simulink model "Slide_SLIPControl_Uneven"  (R2020b)
settings: Solver=VariableStepAuto  StartTime=0.0  StopTime=10  FixedStep=0.01  RelTol=1e-3
undefined symbols (not defined in the file or in its folder): B, Feet, T1, T10, T11, T2, T3, T4, T5, T6, T7, T8, T9, Thigh, Torso, X, Y, Z
libraries: sm_lib x159, nesl_utility x22, simulink x1
(part 1 of 3)
settings Model: Creator=chainplain  LastModifiedBy=chainplain

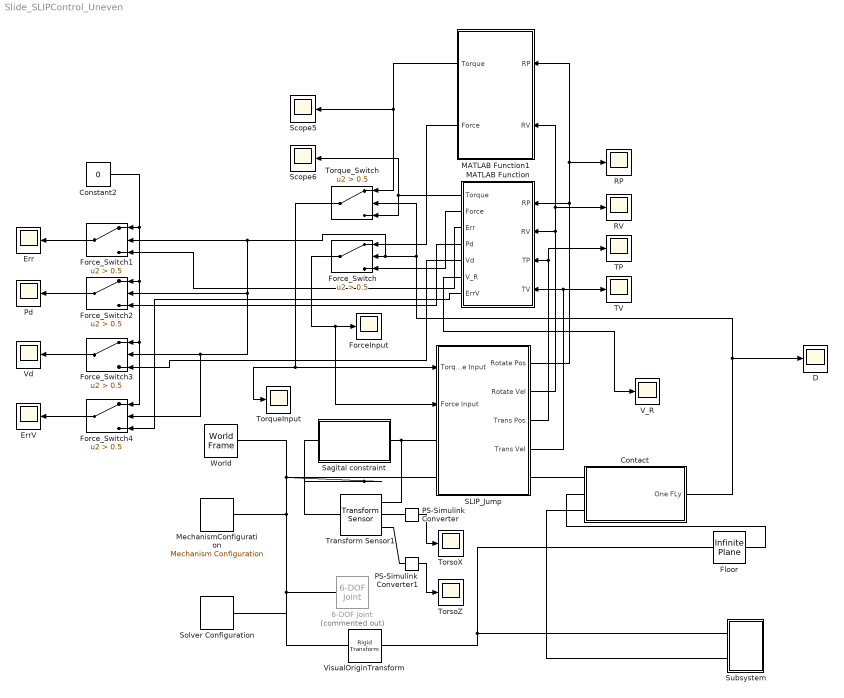
== system Slide_SLIPControl_Uneven ==
  6-DOF Joint : sm_lib/Joints/6-DOF Joint  Commented=on  JointMode=Normal  SenseConstraintForce=off  SenseConstraintForceX=off  SenseConstraintForceY=off  SenseConstraintForceZ=off  SenseConstraintTorque=off  SenseConstraintTorqueX=off  SenseConstraintTorqueY=off  SenseConstraintTorqueZ=off  SenseTotalForce=off  SenseTotalForceX=off  SenseTotalForceY=off  SenseTotalForceZ=off  SenseTotalTorque=off  SenseTotalTorqueX=off  SenseTotalTorqueY=off  SenseTotalTorqueZ=off  CompositeWrenchDir=FollowerOnBase  CompositeWrenchFrame=BaseFrame  PxEquilibriumPosition=0  PxEquilibriumPositionUnits=m  PxSpringStiffness=0  PxSpringStiffnessUnits=N/m  PxDampingCoefficient=0  PxDampingCoefficientUnits=N/(m/s)  PxTorqueActuationMode=NoTorque  PxMotionActuationMode=ComputedMotion  PxSensePosition=off  PxSenseVelocity=off  PxSenseAcceleration=off  PxSenseTorqueForce=off  PxSenseLowerLimitTorqueForce=off  PxSenseUpperLimitTorqueForce=off  PxLowerLimitSpecify=off  PxLowerLimitBound=-1  PxLowerLimitBoundUnits=m  PxLowerLimitStiffness=1e6  PxLowerLimitStiffnessUnits=N/m  PxLowerLimitDamping=1e3  PxLowerLimitDampingUnits=N/(m/s)  PxLowerLimitTransitionRegionWidth=1e-4  PxLowerLimitTransitionRegionWidthUnits=m  PxUpperLimitSpecify=off  PxUpperLimitBound=1  PxUpperLimitBoundUnits=m  PxUpperLimitStiffness=1e6  PxUpperLimitStiffnessUnits=N/m  PxUpperLimitDamping=1e3  PxUpperLimitDampingUnits=N/(m/s)  PxUpperLimitTransitionRegionWidth=1e-4  PxUpperLimitTransitionRegionWidthUnits=m  PxPositionTargetSpecify=off  PxPositionTargetPriority=High  PxPositionTargetValue=0  PxPositionTargetValueUnits=m  PxVelocityTargetSpecify=off  PxVelocityTargetPriority=High  PxVelocityTargetValue=0  PxVelocityTargetValueUnits=m/s  PyEquilibriumPosition=0  PyEquilibriumPositionUnits=m  PySpringStiffness=0  PySpringStiffnessUnits=N/m  PyDampingCoefficient=0  PyDampingCoefficientUnits=N/(m/s)  PyTorqueActuationMode=NoTorque  PyMotionActuationMode=ComputedMotion  PySensePosition=off  PySenseVelocity=off  PySenseAcceleration=off  PySenseTorqueForce=off  PySenseLowerLimitTorqueForce=off  PySenseUpperLimitTorqueForce=off  PyLowerLimitSpecify=off  PyLowerLimitBound=-1  PyLowerLimitBoundUnits=m  PyLowerLimitStiffness=1e6  PyLowerLimitStiffnessUnits=N/m  PyLowerLimitDamping=1e3  PyLowerLimitDampingUnits=N/(m/s)  PyLowerLimitTransitionRegionWidth=1e-4  PyLowerLimitTransitionRegionWidthUnits=m  PyUpperLimitSpecify=off  PyUpperLimitBound=1  PyUpperLimitBoundUnits=m  PyUpperLimitStiffness=1e6  PyUpperLimitStiffnessUnits=N/m  PyUpperLimitDamping=1e3  PyUpperLimitDampingUnits=N/(m/s)  PyUpperLimitTransitionRegionWidth=1e-4  PyUpperLimitTransitionRegionWidthUnits=m  PyPositionTargetSpecify=off  PyPositionTargetPriority=High  PyPositionTargetValue=0  PyPositionTargetValueUnits=m  PyVelocityTargetSpecify=off  PyVelocityTargetPriority=High  PyVelocityTargetValue=0  PyVelocityTargetValueUnits=m/s  PzEquilibriumPosition=0  PzEquilibriumPositionUnits=m  PzSpringStiffness=0  PzSpringStiffnessUnits=N/m  PzDampingCoefficient=0  PzDampingCoefficientUnits=N/(m/s)  PzTorqueActuationMode=NoTorque  PzMotionActuationMode=ComputedMotion  PzSensePosition=off  PzSenseVelocity=off  PzSenseAcceleration=off  PzSenseTorqueForce=off  PzSenseLowerLimitTorqueForce=off  PzSenseUpperLimitTorqueForce=off  PzLowerLimitSpecify=off  PzLowerLimitBound=-1  PzLowerLimitBoundUnits=m  PzLowerLimitStiffness=1e6  PzLowerLimitStiffnessUnits=N/m  PzLowerLimitDamping=1e3  PzLowerLimitDampingUnits=N/(m/s)  PzLowerLimitTransitionRegionWidth=1e-4  PzLowerLimitTransitionRegionWidthUnits=m  PzUpperLimitSpecify=off  PzUpperLimitBound=1  PzUpperLimitBoundUnits=m  PzUpperLimitStiffness=1e6  PzUpperLimitStiffnessUnits=N/m  PzUpperLimitDamping=1e3  PzUpperLimitDampingUnits=N/(m/s)  PzUpperLimitTransitionRegionWidth=1e-4  PzUpperLimitTransitionRegionWidthUnits=m  PzPositionTargetSpecify=off  PzPositionTargetPriority=High  PzPositionTargetValue=0  PzPositionTargetValueUnits=m  PzVelocityTargetSpecify=off  PzVelocityTargetPriority=High  PzVelocityTargetValue=0  PzVelocityTargetValueUnits=m/s  SphDefPosRotationMethod=None  SphDefPosRotationAngleUnits=deg  SphDefPosRotationStandardAxis=+Z  SphDefPosRotationAngle=0.0  SphDefPosRotationArbitraryAxis=[0 0 1]  SphDefPosFollAlignAxisA=+X  SphDefPosBaseAlignAxisA=+Y  SphDefPosFollAlignAxisB=+Y  SphDefPosBaseAlignAxisB=+Z  SphDefPosRotationSequenceAxes=FollowerAxes  SphDefPosRotationSequence=XYX  SphDefPosRotationSequenceAngles=[0 0 0]  SphDefPosRotationSequenceAnglesUnits=deg  SphDefPosRotationMatrix=[1 0 0; 0 1 0; 0 0 1]  SphEqPosRotationMethod=None  SphEqPosRotationAngleUnits=deg  SphEqPosRotationStandardAxis=+Z  SphEqPosRotationAngle=0.0  SphEqPosRotationArbitraryAxis=[0 0 1]  SphEqPosFollAlignAxisA=+X  SphEqPosBaseAlignAxisA=+Y  SphEqPosFollAlignAxisB=+Y  SphEqPosBaseAlignAxisB=+Z  SphEqPosRotationSequenceAxes=FollowerAxes  SphEqPosRotationSequence=XYX  SphEqPosRotationSequenceAngles=[0 0 0]  SphEqPosRotationSequenceAnglesUnits=deg  SphEqPosRotationMatrix=[1 0 0; 0 1 0; 0 0 1]  SphSpringStiffness=0  SphSpringStiffnessUnits=N*m/deg  SphDampingCoefficient=0  SphDampingCoefficientUnits=N*m/(deg/s)  SphActuateTorqueX=off  SphActuateTorqueY=off  SphActuateTorqueZ=off  SphActuateTorque=off  SphTorqueActuationMode=NoTorque  SphMotionActuationMode=ComputedMotion  SphActuationFrame=BaseFrame  SphSensePosition=off  SphSenseVelocityX=off  SphSenseVelocityY=off  SphSenseVelocityZ=off  SphSenseVelocity=off  SphSenseAccelerationX=off  SphSenseAccelerationY=off  SphSenseAccelerationZ=off  SphSenseAcceleration=off  SphSenseTorqueX=off  SphSenseTorqueY=off  SphSenseTorqueZ=off  SphSenseTorqueForce=off  SphSenseLowerLimitTorqueMag=off  SphSenseUpperLimitTorqueMag=off  SphSensingFrame=BaseFrame  SphLowerLimitSpecify=off  SphLowerLimitBound=15  SphLowerLimitBoundUnits=deg  SphLowerLimitStiffness=1e4  SphLowerLimitStiffnessUnits=N*m/deg  SphLowerLimitDamping=10  SphLowerLimitDampingUnits=N*m/(deg/s)  SphLowerLimitTransitionRegionWidth=0.1  SphLowerLimitTransitionRegionWidthUnits=deg  SphUpperLimitSpecify=off  SphUpperLimitBound=45  SphUpperLimitBoundUnits=deg  SphUpperLimitStiffness=1e4  SphUpperLimitStiffnessUnits=N*m/deg  SphUpperLimitDamping=10  SphUpperLimitDampingUnits=N*m/(deg/s)  SphUpperLimitTransitionRegionWidth=0.1  SphUpperLimitTransitionRegionWidthUnits=deg  SphPositionTargetRotationMethod=None  SphPositionTargetRotationAngleUnits=deg  SphPositionTargetRotationStandardAxis=+Z  SphPositionTargetRotationAngle=0.0  SphPositionTargetRotationArbitraryAxis=[0 0 1]  SphPositionTargetFollAlignAxisA=+X  SphPositionTargetBaseAlignAxisA=+Y  SphPositionTargetFollAlignAxisB=+Y  SphPositionTargetBaseAlignAxisB=+Z  SphPositionTargetRotationSequenceAxes=FollowerAxes  SphPositionTargetRotationSequence=XYX  SphPositionTargetRotationSequenceAngles=[0 0 0]  SphPositionTargetRotationSequenceAnglesUnits=deg  SphPositionTargetRotationMatrix=[1 0 0; 0 1 0; 0 0 1]  SphPositionTargetSpecify=off  SphPositionTargetPriority=High  SphVelocityTargetValue=[0 0 0]  SphVelocityTargetValueUnits=deg/s  SphVelocityTargetSpecify=off  SphVelocityTargetPriority=High  SphVelocityTargetInFollowerFrame=on
  Constant2 : Constant  Value=0
  Contact : Subsystem  mask{Stiff=1e6, Damp=1e3, Trans=1e-4, StaticF=0.750, DynamicF=0.500, CriticalV=1e-4}
      mask prompts: Stiff "Contact Stiffness"; Damp "Contact Damping"; Trans "Contact TransRegion"; StaticF "Contact Static Friction"; DynamicF "Contact Dynamic Friction"; CriticalV "Contact Critical Velocity"
      mask DialogControl ContactGroupVar Prompt: Contact
  D : Scope
  Err : Scope
  ErrV : Scope
  Floor : sm_lib/Curves and Surfaces/Infinite Plane  GraphicType=Rectangle  GraphicPlaneWidth=100  GraphicPlaneWidthUnits=m  GraphicPlaneHeight=1  GraphicPlaneHeightUnits=m  GraphicVisPropType=SimpleVisualProperties  GraphicDiffuseColor=[0.5 0.5 0.5]  GraphicOpacity=1  GraphicSpecularColor=[0.5 0.5 0.5 1.0]  GraphicAmbientColor=[0.15 0.15 0.15 1.0]  GraphicEmissiveColor=[0.0 0.0 0.0 1.0]  GraphicShininess=75
  ForceInput : Scope
  Force_Switch{,1..4} (5 alike) : Switch  Criteria=u2 > Threshold  Threshold=0.5
  MATLAB Function : MATLAB Function  TreatAsAtomicUnit=on
  MATLAB Function1 : MATLAB Function  TreatAsAtomicUnit=on
  MechanismConfiguration : sm_lib/Utilities/Mechanism Configuration  UniformGravity=Constant  GravityVector=[0 0 -9.80665]  GravityVectorUnits=m/s^2  GravityUnits=m/s^2  LinearizationDelta=0.001  JointModeTransitionNonlinearIterations=2
  PS-Simulink Converter : nesl_utility/PS-Simulink Converter  PhysicalDomain=network_engine_domain  SubClassName=ps_output  LeftPortType=input  RightPortType=output  PseudoPeriodic=off  Frequencies=[]  Unit=inherit  AffineConversion=off
  PS-Simulink Converter1 : nesl_utility/PS-Simulink Converter  PhysicalDomain=network_engine_domain  SubClassName=ps_output  LeftPortType=input  RightPortType=output  PseudoPeriodic=off  Frequencies=[]  Unit=inherit  AffineConversion=off
  Pd : Scope
  RP : Scope
  RV : Scope
  SLIP_Jump : Subsystem
      mask Display: image('SlipFig.png'); % Use "Edit Image" on toolstrip to change.
  Sagital constraint : Subsystem
  Scope5 : Scope
  Scope6 : Scope
  Solver Configuration : nesl_utility/Solver Configuration  PhysicalDomain=network_engine_domain  SubClassName=solver  LeftPortType=input  RightPortType=generic  Tones=[]  Harmonics=[]  SimulateNoise=off  Profile=off  UseLocalSampling=off  EnableSwitchedLinearOptims=on  FrequencyDomain=off  UseCCode=off  RelTol=0.001  AbsTol=1e-06  MinStep=1e-09  ToWorkspace=off  RevertToSquareIcSolve=off  NumHomotopyIterations=100  PhasorMode=off  PhasorModeNumHarmonics=1  DoDC=off  ResidualTolerance=1e-09  UseLocalSolver=off  LocalSolverChoice=NE_BACKWARD_EULER_ADVANCER  LocalSolverSampleTime=0.001  DoFixedCost=off  MaxNonlinIter=3  MaxModeIter=2  ComputeImpulses=off  ImpulseIterations=2  LinearAlgebra=auto  EquationFormulation=NE_TIME_EF  DelaysMemoryBudget=1024  AutomaticFiltering=on  FilteringTimeConstant=0.001  PartitionStorageMethod=AS_NEEDED  PartitionMemoryBudget=1024  PartitionMethod=ROBUST
  Subsystem : Subsystem
  TP : Scope
  TV : Scope
  TorqueInput : Scope
  Torque_Switch : Switch  Criteria=u2 > Threshold  Threshold=0.5
  TorsoX : Scope
  TorsoZ : Scope
  Transform Sensor1 : sm_lib/Frames and Transforms/Transform Sensor  MeasurementFrame=World  SenseAngle=off  SenseAxis=off  SenseAngle1=off  SenseAngle2=off  SenseAngle3=off  SenseQ=off  SenseR=off  SenseOmegaX=off  SenseOmegaY=off  SenseOmegaZ=off  SenseOmega1=off  SenseOmega2=off  SenseOmega3=off  SenseQDot=off  SenseRDot=off  SenseAlphaX=off  SenseAlphaY=off  SenseAlphaZ=off  SenseAlpha1=off  SenseAlpha2=off  SenseAlpha3=off  SenseQDDot=off  SenseRDDot=off  SenseX=on  SenseY=off  SenseZ=on  SenseRad=off  SenseAzim=off  SenseDist=off  SenseInc=off  SenseXDot=off  SenseYDot=off  SenseZDot=off  SenseRadDot=off  SenseAzimDot=off  SenseDistDot=off  SenseIncDot=off  SenseXDDot=off  SenseYDDot=off  SenseZDDot=off  SenseRadDDot=off  SenseAzimDDot=off  SenseDistDDot=off  SenseIncDDot=off
  V_R : Scope
  Vd : Scope
  VisualOriginTransform : sm_lib/Frames and Transforms/Rigid Transform  TranslationMethod=Cartesian  TranslationStandardOffset=0  TranslationLengthUnit=m  TranslationStandardAxis=+Z  TranslationCartesianOffset=[0, 0.3, -0.7]  TranslationROffset=0  TranslationROffsetUnits=m  TranslationZOffset=0  TranslationZOffsetUnits=m  TranslationThetaOffset=0  TranslationThetaOffsetUnits=deg  RotationMethod=RotationSequence  RotationAngleUnits=deg  RotationStandardAxis=+Z  RotationAngle=0.0  RotationArbitraryAxis=[0 0 1]  FollAlignAxisA=+X  BaseAlignAxisA=+Y  FollAlignAxisB=+Y  BaseAlignAxisB=+Z  RotationSequenceAxes=BaseAxes  RotationSequence=XYZ  RotationSequenceAngles=[0, 0, 0]  RotationSequenceAnglesUnits=rad  RotationMatrix=[1 0 0; 0 1 0; 0 0 1]
  World : sm_lib/Frames and Transforms/World Frame
  wires:
  SLIP_Jump/1(Rotate Pos) -> RP/1, MATLAB Function1/1(RP), MATLAB Function/1(RP)
  SLIP_Jump/2(Rotate Vel) -> RV/1, MATLAB Function1/2(RV), MATLAB Function/2(RV)
  SLIP_Jump/3(Trans Pos) -> TP/1, MATLAB Function/3(TP)
  SLIP_Jump/4(Trans Vel) -> TV/1, MATLAB Function/4(TV)
  MATLAB Function1/1(Torque) -> Torque_Switch/1, Scope5/1
  MATLAB Function1/2(Force) -> Force_Switch/1
  Force_Switch/1 -> SLIP_Jump/2(Force Input), ForceInput/1
  Torque_Switch/1 -> TorqueInput/1, SLIP_Jump/1(Torque Input)
  MATLAB Function/1(Torque) -> Scope6/1, Torque_Switch/3
  MATLAB Function/2(Force) -> Force_Switch/3
  MATLAB Function/3(Err) -> Force_Switch1/3
  Constant2/1 -> Force_Switch4/1, Force_Switch3/1, Force_Switch2/1, Force_Switch1/1
  Force_Switch1/1 -> Err/1
  MATLAB Function/4(Pd) -> Force_Switch2/3
  Contact/1(One FLy) -> Force_Switch4/2, Force_Switch3/2, Force_Switch2/2, Force_Switch1/2, Force_Switch/2, Torque_Switch/2, D/1
  Force_Switch2/1 -> Pd/1
  Force_Switch3/1 -> Vd/1
  Force_Switch4/1 -> ErrV/1
  MATLAB Function/5(Vd) -> Force_Switch3/3
  MATLAB Function/7(ErrV) -> Force_Switch4/3
  PS-Simulink Converter/1 -> TorsoX/1
  PS-Simulink Converter1/1 -> TorsoZ/1
  MATLAB Function/6(V_R) -> V_R/1
  connections:
  MechanismConfiguration/RConn1 -- Transform Sensor1/LConn1 -- Sagital constraint/LConn1 -- World/RConn1 -- SLIP_Jump/LConn2 -- VisualOriginTransform/LConn1 -- Solver Configuration/RConn1 -- 6-DOF Joint/LConn1
  VisualOriginTransform/RConn1 -- Floor/LConn1 -- Subsystem/LConn1
  SLIP_Jump/RConn1 -- Contact/LConn1
  Contact/LConn2 -- Floor/RConn1
  Sagital constraint/RConn1 -- Transform Sensor1/RConn1 -- SLIP_Jump/LConn1
  Contact/LConn3 -- Subsystem/LConn2
  PS-Simulink Converter/LConn1 -- Transform Sensor1/RConn2
  Transform Sensor1/RConn3 -- PS-Simulink Converter1/LConn1

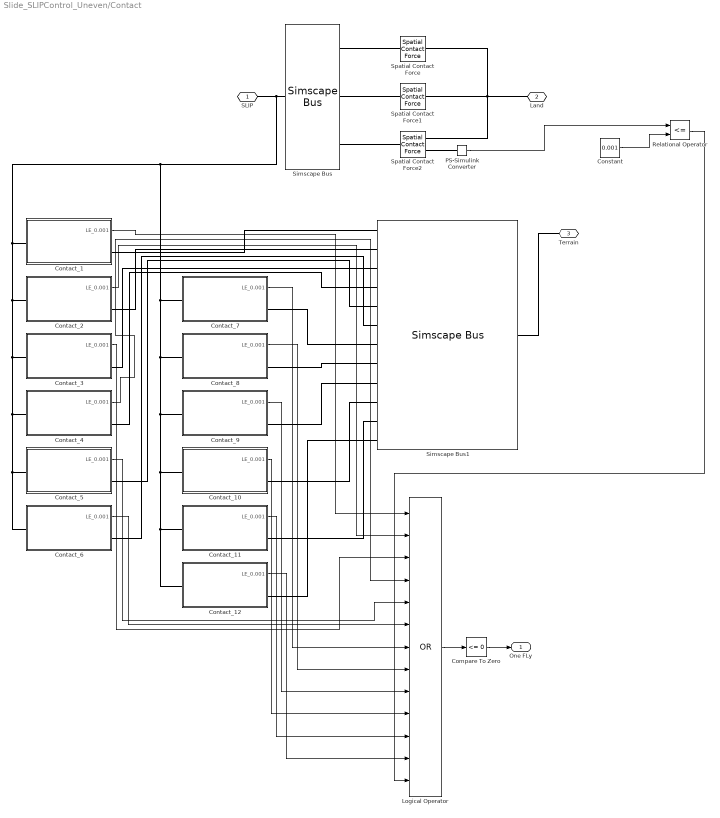
== system Slide_SLIPControl_Uneven/Contact ==
  Compare To Zero : simulink/Logic and Bit Operations/Compare To Zero  relop=<=  OutDataTypeStr=boolean
  Constant : Constant  Value=0.001
  Contact_1 : Subsystem
  Contact_10 : Subsystem
  Contact_11 : Subsystem
  Contact_12 : Subsystem
  Contact_2 : Subsystem
  Contact_3 : Subsystem
  Contact_4 : Subsystem
  Contact_5 : Subsystem
  Contact_6 : Subsystem
  Contact_7 : Subsystem
  Contact_8 : Subsystem
  Contact_9 : Subsystem
  Logical Operator : Logic  Operator=OR  Inputs=13  AllPortsSameDT=off  OutDataTypeStr=boolean
  PS-Simulink Converter : nesl_utility/PS-Simulink Converter  PhysicalDomain=network_engine_domain  SubClassName=ps_output  LeftPortType=input  RightPortType=output  PseudoPeriodic=off  Frequencies=[]  Unit=inherit  AffineConversion=off
  Relational Operator : RelationalOperator  Operator=<=  OutDataTypeStr=boolean  RndMeth=Simplest
  Simscape Bus : SimscapeBus  HierarchyStrings=Torso;Thigh;Feet
  Simscape Bus1 : SimscapeBus  HierarchyStrings=B;T1;T2;T3;T4;T5;T6;T7;T8;T9;T10;T11
  Spatial Contact Force : sm_lib/Forces and Torques/Spatial Contact Force  CoefficientOfDynamicFriction=DynamicF  CoefficientOfStaticFriction=StaticF  NormalDamping=Damp  NormalDampingUnits=N/(m/s)  NormalStiffness=Stiff  NormalStiffnessUnits=N/m  FrictionalCriticalVelocity=CriticalV  FrictionalCriticalVelocityUnits=m/s  ZeroCrossDetectContactStartAndEnd=off  SenseFrictionalForceMagnitude=off  SenseNormalForceMagnitude=off  SenseSeparationDistance=off  NormalTransitionRegionWidth=Trans  NormalTransitionRegionWidthUnits=m  FrictionType=SmoothStickSlip
  Spatial Contact Force1 : sm_lib/Forces and Torques/Spatial Contact Force  CoefficientOfDynamicFriction=DynamicF  CoefficientOfStaticFriction=StaticF  NormalDamping=Damp  NormalDampingUnits=N/(m/s)  NormalStiffness=Stiff  NormalStiffnessUnits=N/m  FrictionalCriticalVelocity=CriticalV  FrictionalCriticalVelocityUnits=m/s  ZeroCrossDetectContactStartAndEnd=off  SenseFrictionalForceMagnitude=off  SenseNormalForceMagnitude=off  SenseSeparationDistance=off  NormalTransitionRegionWidth=Trans  NormalTransitionRegionWidthUnits=m  FrictionType=SmoothStickSlip
  Spatial Contact Force2 : sm_lib/Forces and Torques/Spatial Contact Force  CoefficientOfDynamicFriction=DynamicF  CoefficientOfStaticFriction=StaticF  NormalDamping=Damp  NormalDampingUnits=N/(m/s)  NormalStiffness=Stiff  NormalStiffnessUnits=N/m  FrictionalCriticalVelocity=CriticalV  FrictionalCriticalVelocityUnits=m/s  ZeroCrossDetectContactStartAndEnd=off  SenseFrictionalForceMagnitude=off  SenseNormalForceMagnitude=off  SenseSeparationDistance=on  NormalTransitionRegionWidth=Trans  NormalTransitionRegionWidthUnits=m  FrictionType=SmoothStickSlip
  SLIP : PMIOPort  Side=Left
  Land : PMIOPort  Port=2  Side=Left
  Terrain : PMIOPort  Port=3  Side=Left
  One FLy : Outport
  wires:
  Contact_1/1(LE_0.001) -> Logical Operator/1
  Contact_2/1(LE_0.001) -> Logical Operator/2
  Contact_3/1(LE_0.001) -> Logical Operator/3
  Contact_4/1(LE_0.001) -> Logical Operator/4
  Contact_5/1(LE_0.001) -> Logical Operator/5
  Contact_6/1(LE_0.001) -> Logical Operator/6
  Contact_7/1(LE_0.001) -> Logical Operator/7
  Contact_8/1(LE_0.001) -> Logical Operator/8
  Contact_9/1(LE_0.001) -> Logical Operator/9
  Contact_10/1(LE_0.001) -> Logical Operator/10
  Contact_11/1(LE_0.001) -> Logical Operator/11
  Contact_12/1(LE_0.001) -> Logical Operator/12
  Relational Operator/1 -> Logical Operator/13
  PS-Simulink Converter/1 -> Relational Operator/1
  Constant/1 -> Relational Operator/2
  Compare To Zero/1 -> One FLy/1
  Logical Operator/1 -> Compare To Zero/1
  connections:
  SLIP/RConn1 -- Contact_12/LConn1 -- Contact_11/LConn1 -- Contact_10/LConn1 -- Contact_9/LConn1 -- Contact_8/LConn1 -- Contact_7/LConn1 -- Contact_6/LConn1 -- Contact_5/LConn1 -- Contact_4/LConn1 -- Contact_3/LConn1 -- Contact_2/LConn1 -- Contact_1/LConn1 -- Simscape Bus/RConn1
  Spatial Contact Force/LConn1 -- Simscape Bus/LConn1
  Simscape Bus/LConn2 -- Spatial Contact Force1/LConn1
  Simscape Bus/LConn3 -- Spatial Contact Force2/LConn1
  Spatial Contact Force/RConn1 -- Land/RConn1 -- Spatial Contact Force1/RConn1 -- Spatial Contact Force2/RConn1
  PS-Simulink Converter/LConn1 -- Spatial Contact Force2/RConn2
  Simscape Bus1/RConn1 -- Terrain/RConn1
  Contact_1/RConn1 -- Simscape Bus1/LConn1
  Contact_2/RConn1 -- Simscape Bus1/LConn2
  Contact_3/RConn1 -- Simscape Bus1/LConn3
  Contact_4/RConn1 -- Simscape Bus1/LConn4
  Contact_5/RConn1 -- Simscape Bus1/LConn5
  Contact_6/RConn1 -- Simscape Bus1/LConn6
  Contact_7/RConn1 -- Simscape Bus1/LConn7
  Contact_8/RConn1 -- Simscape Bus1/LConn8
  Contact_9/RConn1 -- Simscape Bus1/LConn9
  Contact_10/RConn1 -- Simscape Bus1/LConn10
  Contact_11/RConn1 -- Simscape Bus1/LConn11
  Contact_12/RConn1 -- Simscape Bus1/LConn12

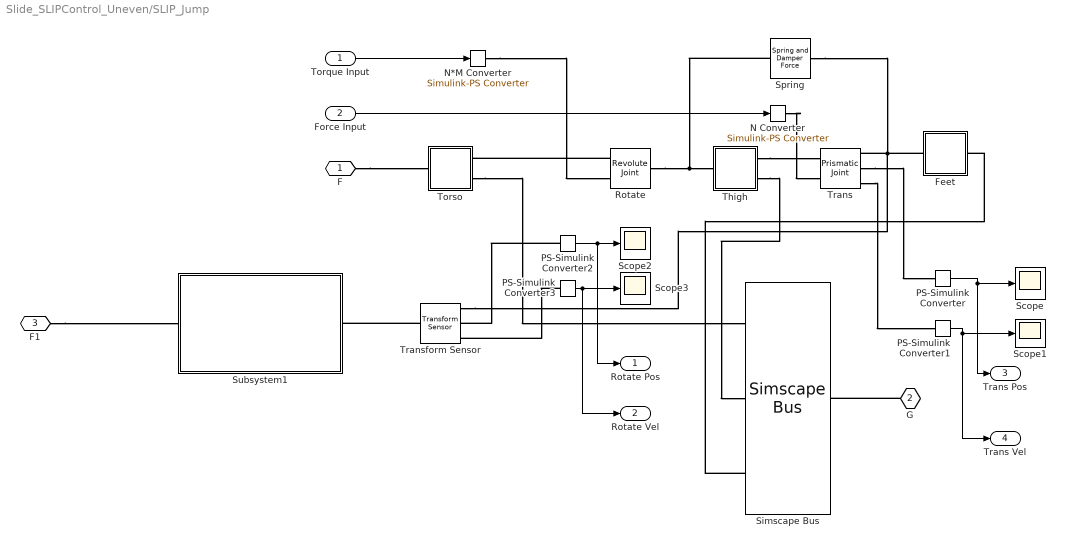
== system Slide_SLIPControl_Uneven/SLIP_Jump ==
  Torque Input : Inport
  Force Input : Inport  Port=2
  Feet : Subsystem
  N Converter : nesl_utility/Simulink-PS Converter  PhysicalDomain=network_engine_domain  SubClassName=ps_input  LeftPortType=input  RightPortType=output  PseudoPeriodic=off  Frequencies=[]  NoiseDistribution=none  NoiseParameters=[]  Unit=N  AffineConversion=off  FilteringAndDerivatives=provide  SimscapeFilterOrder=1  InputFilterTimeConstant=0.001  UdotUserProvided=0
  N*M Converter : nesl_utility/Simulink-PS Converter  PhysicalDomain=network_engine_domain  SubClassName=ps_input  LeftPortType=input  RightPortType=output  PseudoPeriodic=off  Frequencies=[]  NoiseDistribution=none  NoiseParameters=[]  Unit=N*m  AffineConversion=off  FilteringAndDerivatives=provide  SimscapeFilterOrder=1  InputFilterTimeConstant=0.001  UdotUserProvided=0
  PS-Simulink Converter{,1..3} (4 alike) : nesl_utility/PS-Simulink Converter  PhysicalDomain=network_engine_domain  SubClassName=ps_output  LeftPortType=input  RightPortType=output  PseudoPeriodic=off  Frequencies=[]  Unit=inherit  AffineConversion=off
  Rotate : sm_lib/Joints/Revolute Joint  JointMode=Normal  SenseConstraintForce=off  SenseConstraintForceX=off  SenseConstraintForceY=off  SenseConstraintForceZ=off  SenseConstraintTorque=off  SenseConstraintTorqueX=off  SenseConstraintTorqueY=off  SenseConstraintTorqueZ=off  SenseTotalForce=off  SenseTotalForceX=off  SenseTotalForceY=off  SenseTotalForceZ=off  SenseTotalTorque=off  SenseTotalTorqueX=off  SenseTotalTorqueY=off  SenseTotalTorqueZ=off  CompositeWrenchDir=FollowerOnBase  CompositeWrenchFrame=BaseFrame  EquilibriumPosition=0  EquilibriumPositionUnits=deg  SpringStiffness=0  SpringStiffnessUnits=N*m/deg  DampingCoefficient=0  DampingCoefficientUnits=m^2*kg/s/rad  TorqueActuationMode=InputTorque  MotionActuationMode=ComputedMotion  SensePosition=off  SenseVelocity=off  SenseAcceleration=off  SenseTorqueForce=off  SenseLowerLimitTorqueForce=off  SenseUpperLimitTorqueForce=off  LowerLimitSpecify=off  LowerLimitBound=-90  LowerLimitBoundUnits=deg  LowerLimitStiffness=1e4  LowerLimitStiffnessUnits=N*m/deg  LowerLimitDamping=10  LowerLimitDampingUnits=N*m/(deg/s)  LowerLimitTransitionRegionWidth=0.1  LowerLimitTransitionRegionWidthUnits=deg  UpperLimitSpecify=off  UpperLimitBound=90  UpperLimitBoundUnits=deg  UpperLimitStiffness=1e4  UpperLimitStiffnessUnits=N*m/deg  UpperLimitDamping=10  UpperLimitDampingUnits=N*m/(deg/s)  UpperLimitTransitionRegionWidth=0.1  UpperLimitTransitionRegionWidthUnits=deg  PositionTargetSpecify=off  PositionTargetPriority=High  PositionTargetValue=0  PositionTargetValueUnits=deg  VelocityTargetSpecify=off  VelocityTargetPriority=High  VelocityTargetValue=0  VelocityTargetValueUnits=deg/s
  Scope{,1..3} (4 alike) : Scope
  Simscape Bus : SimscapeBus  HierarchyStrings=Torso;Thigh;Feet
  Spring : sm_lib/Forces and Torques/Spring and Damper Force  NaturalLength=0.162  NaturalLengthUnits=m  SpringStiffness=4000  SpringStiffnessUnits=N/m  DampingCoefficient=100  DampingCoefficientUnits=N/(m/s)  SenseForce=off
  Subsystem1 : Subsystem
  Thigh : Subsystem
  Torso : Subsystem
  Trans : sm_lib/Joints/Prismatic Joint  JointMode=Normal  SenseConstraintForce=off  SenseConstraintForceX=off  SenseConstraintForceY=off  SenseConstraintForceZ=off  SenseConstraintTorque=off  SenseConstraintTorqueX=off  SenseConstraintTorqueY=off  SenseConstraintTorqueZ=off  SenseTotalForce=off  SenseTotalForceX=off  SenseTotalForceY=off  SenseTotalForceZ=off  SenseTotalTorque=off  SenseTotalTorqueX=off  SenseTotalTorqueY=off  SenseTotalTorqueZ=off  CompositeWrenchDir=FollowerOnBase  CompositeWrenchFrame=BaseFrame  EquilibriumPosition=0  EquilibriumPositionUnits=m  SpringStiffness=0  SpringStiffnessUnits=N/m  DampingCoefficient=0  DampingCoefficientUnits=kg/s  TorqueActuationMode=InputTorque  MotionActuationMode=ComputedMotion  SensePosition=on  SenseVelocity=on  SenseAcceleration=off  SenseTorqueForce=off  SenseLowerLimitTorqueForce=off  SenseUpperLimitTorqueForce=off  LowerLimitSpecify=on  LowerLimitBound=-0.1  LowerLimitBoundUnits=m  LowerLimitStiffness=1e6  LowerLimitStiffnessUnits=N/m  LowerLimitDamping=1e3  LowerLimitDampingUnits=N/(m/s)  LowerLimitTransitionRegionWidth=1e-4  LowerLimitTransitionRegionWidthUnits=m  UpperLimitSpecify=on  UpperLimitBound=0.02  UpperLimitBoundUnits=m  UpperLimitStiffness=1e6  UpperLimitStiffnessUnits=N/m  UpperLimitDamping=1e3  UpperLimitDampingUnits=N/(m/s)  UpperLimitTransitionRegionWidth=1e-4  UpperLimitTransitionRegionWidthUnits=m  PositionTargetSpecify=off  PositionTargetPriority=High  PositionTargetValue=0  PositionTargetValueUnits=m  VelocityTargetSpecify=off  VelocityTargetPriority=High  VelocityTargetValue=0  VelocityTargetValueUnits=m/s
  Transform Sensor : sm_lib/Frames and Transforms/Transform Sensor  MeasurementFrame=Base  SenseAngle=on  SenseAxis=off  SenseAngle1=off  SenseAngle2=off  SenseAngle3=off  SenseQ=off  SenseR=off  SenseOmegaX=on  SenseOmegaY=off  SenseOmegaZ=off  SenseOmega1=off  SenseOmega2=off  SenseOmega3=off  SenseQDot=off  SenseRDot=off  SenseAlphaX=off  SenseAlphaY=off  SenseAlphaZ=off  SenseAlpha1=off  SenseAlpha2=off  SenseAlpha3=off  SenseQDDot=off  SenseRDDot=off  SenseX=off  SenseY=off  SenseZ=off  SenseRad=off  SenseAzim=off  SenseDist=off  SenseInc=off  SenseXDot=off  SenseYDot=off  SenseZDot=off  SenseRadDot=off  SenseAzimDot=off  SenseDistDot=off  SenseIncDot=off  SenseXDDot=off  SenseYDDot=off  SenseZDDot=off  SenseRadDDot=off  SenseAzimDDot=off  SenseDistDDot=off  SenseIncDDot=off
  F : PMIOPort  Side=Left
  G : PMIOPort  Port=2  Side=Right
  F1 : PMIOPort  Port=3  Side=Left
  Rotate Pos : Outport
  Rotate Vel : Outport  Port=2
  Trans Pos : Outport  Port=3
  Trans Vel : Outport  Port=4
  wires:
  Force Input/1 -> N Converter/1
  PS-Simulink Converter/1 -> Trans Pos/1, Scope/1
  Torque Input/1 -> N*M Converter/1
  PS-Simulink Converter1/1 -> Trans Vel/1, Scope1/1
  PS-Simulink Converter2/1 -> Rotate Pos/1, Scope2/1
  PS-Simulink Converter3/1 -> Rotate Vel/1, Scope3/1
  connections:
  Thigh/RConn1 -- Trans/LConn1
  Feet/LConn1 -- Trans/RConn1 -- Spring/RConn1 -- Transform Sensor/RConn1
  Rotate/RConn1 -- Spring/LConn1 -- Thigh/LConn1
  Rotate/LConn1 -- Torso/RConn1
  F/RConn1 -- Torso/LConn1
  G/RConn1 -- Simscape Bus/RConn1
  Torso/RConn2 -- Simscape Bus/LConn1
  Thigh/RConn2 -- Simscape Bus/LConn2
  Simscape Bus/LConn3 -- Feet/RConn1
  N*M Converter/RConn1 -- Rotate/LConn2
  N Converter/RConn1 -- Trans/LConn2
  Trans/RConn2 -- PS-Simulink Converter/LConn1
  Trans/RConn3 -- PS-Simulink Converter1/LConn1
  F1/RConn1 -- Subsystem1/LConn1
  Transform Sensor/LConn1 -- Subsystem1/RConn1
  PS-Simulink Converter2/LConn1 -- Transform Sensor/RConn2
  PS-Simulink Converter3/LConn1 -- Transform Sensor/RConn3

== system Slide_SLIPControl_Uneven/Sagital constraint ==
  Infinite Plane1 : sm_lib/Curves and Surfaces/Infinite Plane  GraphicType=Rectangle  GraphicPlaneWidth=1  GraphicPlaneWidthUnits=m  GraphicPlaneHeight=1  GraphicPlaneHeightUnits=m  GraphicVisPropType=SimpleVisualProperties  GraphicDiffuseColor=[0.5 0.5 0.5]  GraphicOpacity=0.1  GraphicSpecularColor=[0.5 0.5 0.5 1.0]  GraphicAmbientColor=[0.15 0.15 0.15 1.0]  GraphicEmissiveColor=[0.0 0.0 0.0 1.0]  GraphicShininess=75
  Rectangular Joint : sm_lib/Joints/Rectangular Joint  JointMode=Normal  SenseConstraintForce=off  SenseConstraintForceX=off  SenseConstraintForceY=off  SenseConstraintForceZ=off  SenseConstraintTorque=off  SenseConstraintTorqueX=off  SenseConstraintTorqueY=off  SenseConstraintTorqueZ=off  SenseTotalForce=off  SenseTotalForceX=off  SenseTotalForceY=off  SenseTotalForceZ=off  SenseTotalTorque=off  SenseTotalTorqueX=off  SenseTotalTorqueY=off  SenseTotalTorqueZ=off  CompositeWrenchDir=FollowerOnBase  CompositeWrenchFrame=BaseFrame  PxEquilibriumPosition=0  PxEquilibriumPositionUnits=m  PxSpringStiffness=0  PxSpringStiffnessUnits=N/m  PxDampingCoefficient=0  PxDampingCoefficientUnits=N/(m/s)  PxTorqueActuationMode=NoTorque  PxMotionActuationMode=ComputedMotion  PxSensePosition=off  PxSenseVelocity=off  PxSenseAcceleration=off  PxSenseTorqueForce=off  PxSenseLowerLimitTorqueForce=off  PxSenseUpperLimitTorqueForce=off  PxLowerLimitSpecify=off  PxLowerLimitBound=-1  PxLowerLimitBoundUnits=m  PxLowerLimitStiffness=1e6  PxLowerLimitStiffnessUnits=N/m  PxLowerLimitDamping=1e3  PxLowerLimitDampingUnits=N/(m/s)  PxLowerLimitTransitionRegionWidth=1e-4  PxLowerLimitTransitionRegionWidthUnits=m  PxUpperLimitSpecify=off  PxUpperLimitBound=1  PxUpperLimitBoundUnits=m  PxUpperLimitStiffness=1e6  PxUpperLimitStiffnessUnits=N/m  PxUpperLimitDamping=1e3  PxUpperLimitDampingUnits=N/(m/s)  PxUpperLimitTransitionRegionWidth=1e-4  PxUpperLimitTransitionRegionWidthUnits=m  PxPositionTargetSpecify=off  PxPositionTargetPriority=High  PxPositionTargetValue=0  PxPositionTargetValueUnits=m  PxVelocityTargetSpecify=off  PxVelocityTargetPriority=High  PxVelocityTargetValue=0  PxVelocityTargetValueUnits=m/s  PyEquilibriumPosition=0  PyEquilibriumPositionUnits=m  PySpringStiffness=0  PySpringStiffnessUnits=N/m  PyDampingCoefficient=0  PyDampingCoefficientUnits=N/(m/s)  PyTorqueActuationMode=NoTorque  PyMotionActuationMode=ComputedMotion  PySensePosition=off  PySenseVelocity=off  PySenseAcceleration=off  PySenseTorqueForce=off  PySenseLowerLimitTorqueForce=off  PySenseUpperLimitTorqueForce=off  PyLowerLimitSpecify=off  PyLowerLimitBound=-1  PyLowerLimitBoundUnits=m  PyLowerLimitStiffness=1e6  PyLowerLimitStiffnessUnits=N/m  PyLowerLimitDamping=1e3  PyLowerLimitDampingUnits=N/(m/s)  PyLowerLimitTransitionRegionWidth=1e-4  PyLowerLimitTransitionRegionWidthUnits=m  PyUpperLimitSpecify=off  PyUpperLimitBound=1  PyUpperLimitBoundUnits=m  PyUpperLimitStiffness=1e6  PyUpperLimitStiffnessUnits=N/m  PyUpperLimitDamping=1e3  PyUpperLimitDampingUnits=N/(m/s)  PyUpperLimitTransitionRegionWidth=1e-4  PyUpperLimitTransitionRegionWidthUnits=m  PyPositionTargetSpecify=off  PyPositionTargetPriority=High  PyPositionTargetValue=0  PyPositionTargetValueUnits=m  PyVelocityTargetSpecify=off  PyVelocityTargetPriority=High  PyVelocityTargetValue=0  PyVelocityTargetValueUnits=m/s
  VisualOriginTransform1 : sm_lib/Frames and Transforms/Rigid Transform  TranslationMethod=Cartesian  TranslationStandardOffset=0  TranslationLengthUnit=m  TranslationStandardAxis=+Z  TranslationCartesianOffset=[0, 0, 0]  TranslationROffset=0  TranslationROffsetUnits=m  TranslationZOffset=0  TranslationZOffsetUnits=m  TranslationThetaOffset=0  TranslationThetaOffsetUnits=deg  RotationMethod=RotationSequence  RotationAngleUnits=deg  RotationStandardAxis=+Z  RotationAngle=0.0  RotationArbitraryAxis=[0 0 1]  FollAlignAxisA=+X  BaseAlignAxisA=+Y  FollAlignAxisB=+Y  BaseAlignAxisB=+Z  RotationSequenceAxes=BaseAxes  RotationSequence=XYZ  RotationSequenceAngles="[pi/2,  0, 0]"  RotationSequenceAnglesUnits=rad  RotationMatrix=[1 0 0; 0 1 0; 0 0 1]
  VisualOriginTransform2 : sm_lib/Frames and Transforms/Rigid Transform  TranslationMethod=Cartesian  TranslationStandardOffset=0  TranslationLengthUnit=m  TranslationStandardAxis=+Z  TranslationCartesianOffset=[0, 0, 0]  TranslationROffset=0  TranslationROffsetUnits=m  TranslationZOffset=0  TranslationZOffsetUnits=m  TranslationThetaOffset=0  TranslationThetaOffsetUnits=deg  RotationMethod=RotationSequence  RotationAngleUnits=deg  RotationStandardAxis=+Z  RotationAngle=0.0  RotationArbitraryAxis=[0 0 1]  FollAlignAxisA=+X  BaseAlignAxisA=+Y  FollAlignAxisB=+Y  BaseAlignAxisB=+Z  RotationSequenceAxes=BaseAxes  RotationSequence=XYZ  RotationSequenceAngles="[-pi/2,  pi/2, 0]"  RotationSequenceAnglesUnits=rad  RotationMatrix=[1 0 0; 0 1 0; 0 0 1]
  World : PMIOPort  Side=Left
  ReduWorld : PMIOPort  Port=2  Side=Right
  connections:
  Infinite Plane1/LConn1 -- VisualOriginTransform1/RConn1 -- Rectangular Joint/LConn1
  VisualOriginTransform2/LConn1 -- Rectangular Joint/RConn1
  VisualOriginTransform2/RConn1 -- ReduWorld/RConn1
  VisualOriginTransform1/LConn1 -- World/RConn1

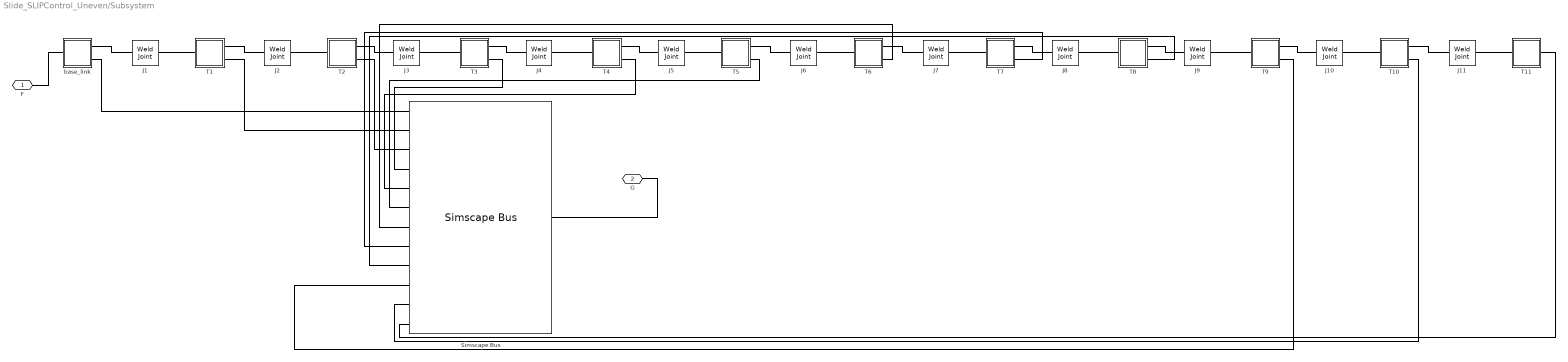
== system Slide_SLIPControl_Uneven/Subsystem ==
  J{1..11} (11 alike) : sm_lib/Joints/Weld Joint  JointMode=Normal  SenseConstraintForce=off  SenseConstraintForceX=off  SenseConstraintForceY=off  SenseConstraintForceZ=off  SenseConstraintTorque=off  SenseConstraintTorqueX=off  SenseConstraintTorqueY=off  SenseConstraintTorqueZ=off  SenseTotalForce=off  SenseTotalForceX=off  SenseTotalForceY=off  SenseTotalForceZ=off  SenseTotalTorque=off  SenseTotalTorqueX=off  SenseTotalTorqueY=off  SenseTotalTorqueZ=off  CompositeWrenchDir=FollowerOnBase  CompositeWrenchFrame=BaseFrame
  Simscape Bus : SimscapeBus  HierarchyStrings=B;T1;T2;T3;T4;T5;T6;T7;T8;T9;T10;T11
  T1 : Subsystem
  T10 : Subsystem
  T11 : Subsystem
  T2 : Subsystem
  T3 : Subsystem
  T4 : Subsystem
  T5 : Subsystem
  T6 : Subsystem
  T7 : Subsystem
  T8 : Subsystem
  T9 : Subsystem
  base_link : Subsystem
  F : PMIOPort  Side=Left
  G : PMIOPort  Port=2  Side=Left
  connections:
  J6/LConn1 -- T5/RConn1
  J4/LConn1 -- T3/RConn1
  J8/RConn1 -- T8/LConn1
  J2/LConn1 -- T1/RConn1
  J1/RConn1 -- T1/LConn1
  J5/LConn1 -- T4/RConn1
  J5/RConn1 -- T5/LConn1
  J7/RConn1 -- T7/LConn1
  J11/LConn1 -- T10/RConn1
  J7/LConn1 -- T6/RConn1
  J8/LConn1 -- T7/RConn1
  J9/RConn1 -- T9/LConn1
  J10/RConn1 -- T10/LConn1
  J6/RConn1 -- T6/LConn1
  J2/RConn1 -- T2/LConn1
  J1/LConn1 -- base_link/RConn1
  J4/RConn1 -- T4/LConn1
  J9/LConn1 -- T8/RConn1
  J3/RConn1 -- T3/LConn1
  J3/LConn1 -- T2/RConn1
  J11/RConn1 -- T11/LConn1
  J10/LConn1 -- T9/RConn1
  F/RConn1 -- base_link/LConn1
  base_link/RConn2 -- Simscape Bus/LConn1
  T1/RConn2 -- Simscape Bus/LConn2
  T2/RConn2 -- Simscape Bus/LConn3
  T3/RConn2 -- Simscape Bus/LConn4
  Simscape Bus/LConn5 -- T4/RConn2
  Simscape Bus/LConn6 -- T5/RConn2
  T6/RConn2 -- Simscape Bus/LConn7
  T7/RConn2 -- Simscape Bus/LConn8
  T8/RConn2 -- Simscape Bus/LConn9
  T9/RConn2 -- Simscape Bus/LConn10
  Simscape Bus/LConn11 -- T10/RConn2
  T11/RConn1 -- Simscape Bus/LConn12
  G/RConn1 -- Simscape Bus/RConn1

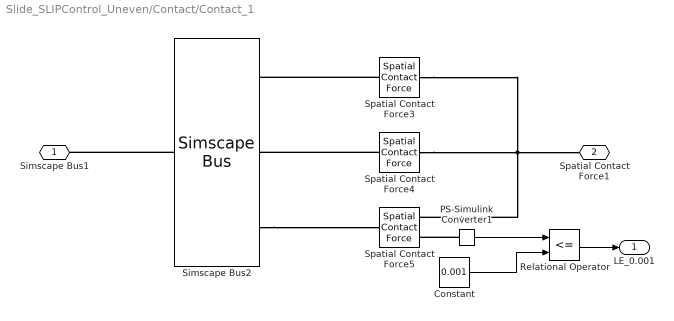
== system Slide_SLIPControl_Uneven/Contact/Contact_1 ==
  Constant : Constant  Value=0.001
  PS-Simulink Converter1 : nesl_utility/PS-Simulink Converter  PhysicalDomain=network_engine_domain  SubClassName=ps_output  LeftPortType=input  RightPortType=output  PseudoPeriodic=off  Frequencies=[]  Unit=inherit  AffineConversion=off
  Relational Operator : RelationalOperator  Operator=<=  OutDataTypeStr=boolean  RndMeth=Simplest
  Simscape Bus2 : SimscapeBus  HierarchyStrings=Torso;Thigh;Feet
  Spatial Contact Force3 : sm_lib/Forces and Torques/Spatial Contact Force  CoefficientOfDynamicFriction=DynamicF  CoefficientOfStaticFriction=StaticF  NormalDamping=Damp  NormalDampingUnits=N/(m/s)  NormalStiffness=Stiff  NormalStiffnessUnits=N/m  FrictionalCriticalVelocity=CriticalV  FrictionalCriticalVelocityUnits=m/s  ZeroCrossDetectContactStartAndEnd=off  SenseFrictionalForceMagnitude=off  SenseNormalForceMagnitude=off  SenseSeparationDistance=off  NormalTransitionRegionWidth=Trans  NormalTransitionRegionWidthUnits=m  FrictionType=SmoothStickSlip
  Spatial Contact Force4 : sm_lib/Forces and Torques/Spatial Contact Force  CoefficientOfDynamicFriction=DynamicF  CoefficientOfStaticFriction=StaticF  NormalDamping=Damp  NormalDampingUnits=N/(m/s)  NormalStiffness=Stiff  NormalStiffnessUnits=N/m  FrictionalCriticalVelocity=CriticalV  FrictionalCriticalVelocityUnits=m/s  ZeroCrossDetectContactStartAndEnd=off  SenseFrictionalForceMagnitude=off  SenseNormalForceMagnitude=off  SenseSeparationDistance=off  NormalTransitionRegionWidth=Trans  NormalTransitionRegionWidthUnits=m  FrictionType=SmoothStickSlip
  Spatial Contact Force5 : sm_lib/Forces and Torques/Spatial Contact Force  CoefficientOfDynamicFriction=DynamicF  CoefficientOfStaticFriction=StaticF  NormalDamping=Damp  NormalDampingUnits=N/(m/s)  NormalStiffness=Stiff  NormalStiffnessUnits=N/m  FrictionalCriticalVelocity=CriticalV  FrictionalCriticalVelocityUnits=m/s  ZeroCrossDetectContactStartAndEnd=off  SenseFrictionalForceMagnitude=off  SenseNormalForceMagnitude=off  SenseSeparationDistance=on  NormalTransitionRegionWidth=Trans  NormalTransitionRegionWidthUnits=m  FrictionType=SmoothStickSlip
  Simscape Bus1 : PMIOPort  Side=Left
  Spatial Contact Force1 : PMIOPort  Port=2  Side=Right
  LE_0.001 : Outport
  wires:
  PS-Simulink Converter1/1 -> Relational Operator/1
  Constant/1 -> Relational Operator/2
  Relational Operator/1 -> LE_0.001/1
  connections:
  Simscape Bus2/LConn3 -- Spatial Contact Force5/LConn1
  Spatial Contact Force3/LConn1 -- Simscape Bus2/LConn1
  Spatial Contact Force4/RConn1 -- Spatial Contact Force1/RConn1 -- Spatial Contact Force5/RConn1 -- Spatial Contact Force3/RConn1
  Simscape Bus2/RConn1 -- Simscape Bus1/RConn1
  Spatial Contact Force4/LConn1 -- Simscape Bus2/LConn2
  PS-Simulink Converter1/LConn1 -- Spatial Contact Force5/RConn2

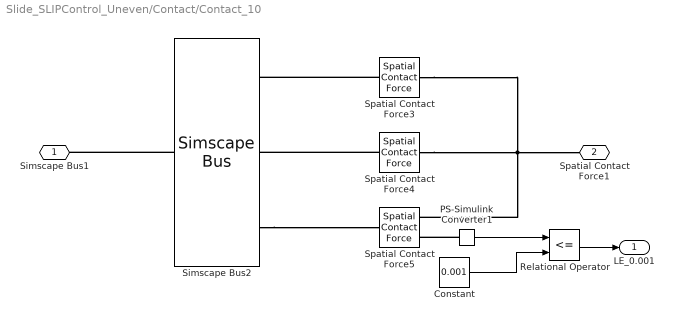
== system Slide_SLIPControl_Uneven/Contact/Contact_10 ==
  Constant : Constant  Value=0.001
  PS-Simulink Converter1 : nesl_utility/PS-Simulink Converter  PhysicalDomain=network_engine_domain  SubClassName=ps_output  LeftPortType=input  RightPortType=output  PseudoPeriodic=off  Frequencies=[]  Unit=inherit  AffineConversion=off
  Relational Operator : RelationalOperator  Operator=<=  OutDataTypeStr=boolean  RndMeth=Simplest
  Simscape Bus2 : SimscapeBus  HierarchyStrings=Torso;Thigh;Feet
  Spatial Contact Force3 : sm_lib/Forces and Torques/Spatial Contact Force  CoefficientOfDynamicFriction=DynamicF  CoefficientOfStaticFriction=StaticF  NormalDamping=Damp  NormalDampingUnits=N/(m/s)  NormalStiffness=Stiff  NormalStiffnessUnits=N/m  FrictionalCriticalVelocity=CriticalV  FrictionalCriticalVelocityUnits=m/s  ZeroCrossDetectContactStartAndEnd=off  SenseFrictionalForceMagnitude=off  SenseNormalForceMagnitude=off  SenseSeparationDistance=off  NormalTransitionRegionWidth=Trans  NormalTransitionRegionWidthUnits=m  FrictionType=SmoothStickSlip
  Spatial Contact Force4 : sm_lib/Forces and Torques/Spatial Contact Force  CoefficientOfDynamicFriction=DynamicF  CoefficientOfStaticFriction=StaticF  NormalDamping=Damp  NormalDampingUnits=N/(m/s)  NormalStiffness=Stiff  NormalStiffnessUnits=N/m  FrictionalCriticalVelocity=CriticalV  FrictionalCriticalVelocityUnits=m/s  ZeroCrossDetectContactStartAndEnd=off  SenseFrictionalForceMagnitude=off  SenseNormalForceMagnitude=off  SenseSeparationDistance=off  NormalTransitionRegionWidth=Trans  NormalTransitionRegionWidthUnits=m  FrictionType=SmoothStickSlip
  Spatial Contact Force5 : sm_lib/Forces and Torques/Spatial Contact Force  CoefficientOfDynamicFriction=DynamicF  CoefficientOfStaticFriction=StaticF  NormalDamping=Damp  NormalDampingUnits=N/(m/s)  NormalStiffness=Stiff  NormalStiffnessUnits=N/m  FrictionalCriticalVelocity=CriticalV  FrictionalCriticalVelocityUnits=m/s  ZeroCrossDetectContactStartAndEnd=off  SenseFrictionalForceMagnitude=off  SenseNormalForceMagnitude=off  SenseSeparationDistance=on  NormalTransitionRegionWidth=Trans  NormalTransitionRegionWidthUnits=m  FrictionType=SmoothStickSlip
  Simscape Bus1 : PMIOPort  Side=Left
  Spatial Contact Force1 : PMIOPort  Port=2  Side=Right
  LE_0.001 : Outport
  wires:
  PS-Simulink Converter1/1 -> Relational Operator/1
  Constant/1 -> Relational Operator/2
  Relational Operator/1 -> LE_0.001/1
  connections:
  Simscape Bus2/LConn3 -- Spatial Contact Force5/LConn1
  Spatial Contact Force3/LConn1 -- Simscape Bus2/LConn1
  Spatial Contact Force4/RConn1 -- Spatial Contact Force1/RConn1 -- Spatial Contact Force5/RConn1 -- Spatial Contact Force3/RConn1
  Simscape Bus2/RConn1 -- Simscape Bus1/RConn1
  Spatial Contact Force4/LConn1 -- Simscape Bus2/LConn2
  PS-Simulink Converter1/LConn1 -- Spatial Contact Force5/RConn2

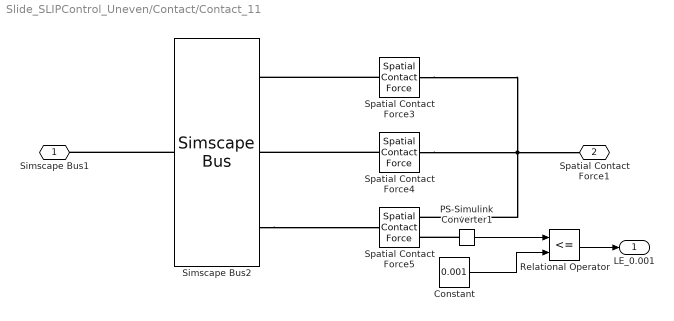
== system Slide_SLIPControl_Uneven/Contact/Contact_11 ==
  Constant : Constant  Value=0.001
  PS-Simulink Converter1 : nesl_utility/PS-Simulink Converter  PhysicalDomain=network_engine_domain  SubClassName=ps_output  LeftPortType=input  RightPortType=output  PseudoPeriodic=off  Frequencies=[]  Unit=inherit  AffineConversion=off
  Relational Operator : RelationalOperator  Operator=<=  OutDataTypeStr=boolean  RndMeth=Simplest
  Simscape Bus2 : SimscapeBus  HierarchyStrings=Torso;Thigh;Feet
  Spatial Contact Force3 : sm_lib/Forces and Torques/Spatial Contact Force  CoefficientOfDynamicFriction=DynamicF  CoefficientOfStaticFriction=StaticF  NormalDamping=Damp  NormalDampingUnits=N/(m/s)  NormalStiffness=Stiff  NormalStiffnessUnits=N/m  FrictionalCriticalVelocity=CriticalV  FrictionalCriticalVelocityUnits=m/s  ZeroCrossDetectContactStartAndEnd=off  SenseFrictionalForceMagnitude=off  SenseNormalForceMagnitude=off  SenseSeparationDistance=off  NormalTransitionRegionWidth=Trans  NormalTransitionRegionWidthUnits=m  FrictionType=SmoothStickSlip
  Spatial Contact Force4 : sm_lib/Forces and Torques/Spatial Contact Force  CoefficientOfDynamicFriction=DynamicF  CoefficientOfStaticFriction=StaticF  NormalDamping=Damp  NormalDampingUnits=N/(m/s)  NormalStiffness=Stiff  NormalStiffnessUnits=N/m  FrictionalCriticalVelocity=CriticalV  FrictionalCriticalVelocityUnits=m/s  ZeroCrossDetectContactStartAndEnd=off  SenseFrictionalForceMagnitude=off  SenseNormalForceMagnitude=off  SenseSeparationDistance=off  NormalTransitionRegionWidth=Trans  NormalTransitionRegionWidthUnits=m  FrictionType=SmoothStickSlip
  Spatial Contact Force5 : sm_lib/Forces and Torques/Spatial Contact Force  CoefficientOfDynamicFriction=DynamicF  CoefficientOfStaticFriction=StaticF  NormalDamping=Damp  NormalDampingUnits=N/(m/s)  NormalStiffness=Stiff  NormalStiffnessUnits=N/m  FrictionalCriticalVelocity=CriticalV  FrictionalCriticalVelocityUnits=m/s  ZeroCrossDetectContactStartAndEnd=off  SenseFrictionalForceMagnitude=off  SenseNormalForceMagnitude=off  SenseSeparationDistance=on  NormalTransitionRegionWidth=Trans  NormalTransitionRegionWidthUnits=m  FrictionType=SmoothStickSlip
  Simscape Bus1 : PMIOPort  Side=Left
  Spatial Contact Force1 : PMIOPort  Port=2  Side=Right
  LE_0.001 : Outport
  wires:
  PS-Simulink Converter1/1 -> Relational Operator/1
  Constant/1 -> Relational Operator/2
  Relational Operator/1 -> LE_0.001/1
  connections:
  Simscape Bus2/LConn3 -- Spatial Contact Force5/LConn1
  Spatial Contact Force3/LConn1 -- Simscape Bus2/LConn1
  Spatial Contact Force4/RConn1 -- Spatial Contact Force1/RConn1 -- Spatial Contact Force5/RConn1 -- Spatial Contact Force3/RConn1
  Simscape Bus2/RConn1 -- Simscape Bus1/RConn1
  Spatial Contact Force4/LConn1 -- Simscape Bus2/LConn2
  PS-Simulink Converter1/LConn1 -- Spatial Contact Force5/RConn2

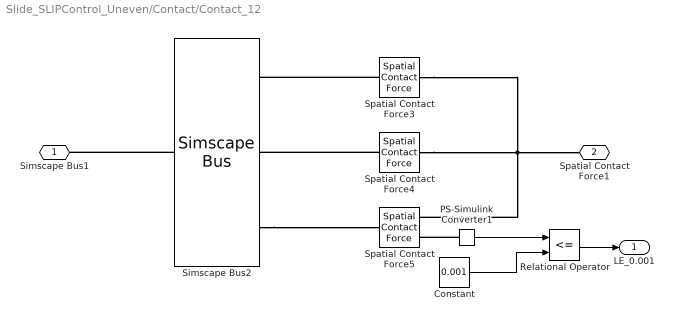
== system Slide_SLIPControl_Uneven/Contact/Contact_12 ==
  Constant : Constant  Value=0.001
  PS-Simulink Converter1 : nesl_utility/PS-Simulink Converter  PhysicalDomain=network_engine_domain  SubClassName=ps_output  LeftPortType=input  RightPortType=output  PseudoPeriodic=off  Frequencies=[]  Unit=inherit  AffineConversion=off
  Relational Operator : RelationalOperator  Operator=<=  OutDataTypeStr=boolean  RndMeth=Simplest
  Simscape Bus2 : SimscapeBus  HierarchyStrings=Torso;Thigh;Feet
  Spatial Contact Force3 : sm_lib/Forces and Torques/Spatial Contact Force  CoefficientOfDynamicFriction=DynamicF  CoefficientOfStaticFriction=StaticF  NormalDamping=Damp  NormalDampingUnits=N/(m/s)  NormalStiffness=Stiff  NormalStiffnessUnits=N/m  FrictionalCriticalVelocity=CriticalV  FrictionalCriticalVelocityUnits=m/s  ZeroCrossDetectContactStartAndEnd=off  SenseFrictionalForceMagnitude=off  SenseNormalForceMagnitude=off  SenseSeparationDistance=off  NormalTransitionRegionWidth=Trans  NormalTransitionRegionWidthUnits=m  FrictionType=SmoothStickSlip
  Spatial Contact Force4 : sm_lib/Forces and Torques/Spatial Contact Force  CoefficientOfDynamicFriction=DynamicF  CoefficientOfStaticFriction=StaticF  NormalDamping=Damp  NormalDampingUnits=N/(m/s)  NormalStiffness=Stiff  NormalStiffnessUnits=N/m  FrictionalCriticalVelocity=CriticalV  FrictionalCriticalVelocityUnits=m/s  ZeroCrossDetectContactStartAndEnd=off  SenseFrictionalForceMagnitude=off  SenseNormalForceMagnitude=off  SenseSeparationDistance=off  NormalTransitionRegionWidth=Trans  NormalTransitionRegionWidthUnits=m  FrictionType=SmoothStickSlip
  Spatial Contact Force5 : sm_lib/Forces and Torques/Spatial Contact Force  CoefficientOfDynamicFriction=DynamicF  CoefficientOfStaticFriction=StaticF  NormalDamping=Damp  NormalDampingUnits=N/(m/s)  NormalStiffness=Stiff  NormalStiffnessUnits=N/m  FrictionalCriticalVelocity=CriticalV  FrictionalCriticalVelocityUnits=m/s  ZeroCrossDetectContactStartAndEnd=off  SenseFrictionalForceMagnitude=off  SenseNormalForceMagnitude=off  SenseSeparationDistance=on  NormalTransitionRegionWidth=Trans  NormalTransitionRegionWidthUnits=m  FrictionType=SmoothStickSlip
  Simscape Bus1 : PMIOPort  Side=Left
  Spatial Contact Force1 : PMIOPort  Port=2  Side=Right
  LE_0.001 : Outport
  wires:
  PS-Simulink Converter1/1 -> Relational Operator/1
  Constant/1 -> Relational Operator/2
  Relational Operator/1 -> LE_0.001/1
  connections:
  Simscape Bus2/LConn3 -- Spatial Contact Force5/LConn1
  Spatial Contact Force3/LConn1 -- Simscape Bus2/LConn1
  Spatial Contact Force4/RConn1 -- Spatial Contact Force1/RConn1 -- Spatial Contact Force5/RConn1 -- Spatial Contact Force3/RConn1
  Simscape Bus2/RConn1 -- Simscape Bus1/RConn1
  Spatial Contact Force4/LConn1 -- Simscape Bus2/LConn2
  PS-Simulink Converter1/LConn1 -- Spatial Contact Force5/RConn2

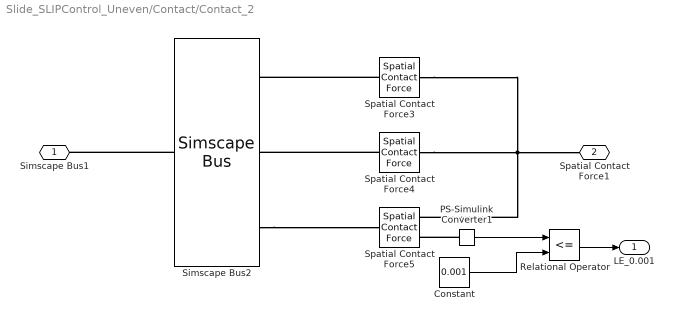
== system Slide_SLIPControl_Uneven/Contact/Contact_2 ==
  Constant : Constant  Value=0.001
  PS-Simulink Converter1 : nesl_utility/PS-Simulink Converter  PhysicalDomain=network_engine_domain  SubClassName=ps_output  LeftPortType=input  RightPortType=output  PseudoPeriodic=off  Frequencies=[]  Unit=inherit  AffineConversion=off
  Relational Operator : RelationalOperator  Operator=<=  OutDataTypeStr=boolean  RndMeth=Simplest
  Simscape Bus2 : SimscapeBus  HierarchyStrings=Torso;Thigh;Feet
  Spatial Contact Force3 : sm_lib/Forces and Torques/Spatial Contact Force  CoefficientOfDynamicFriction=DynamicF  CoefficientOfStaticFriction=StaticF  NormalDamping=Damp  NormalDampingUnits=N/(m/s)  NormalStiffness=Stiff  NormalStiffnessUnits=N/m  FrictionalCriticalVelocity=CriticalV  FrictionalCriticalVelocityUnits=m/s  ZeroCrossDetectContactStartAndEnd=off  SenseFrictionalForceMagnitude=off  SenseNormalForceMagnitude=off  SenseSeparationDistance=off  NormalTransitionRegionWidth=Trans  NormalTransitionRegionWidthUnits=m  FrictionType=SmoothStickSlip
  Spatial Contact Force4 : sm_lib/Forces and Torques/Spatial Contact Force  CoefficientOfDynamicFriction=DynamicF  CoefficientOfStaticFriction=StaticF  NormalDamping=Damp  NormalDampingUnits=N/(m/s)  NormalStiffness=Stiff  NormalStiffnessUnits=N/m  FrictionalCriticalVelocity=CriticalV  FrictionalCriticalVelocityUnits=m/s  ZeroCrossDetectContactStartAndEnd=off  SenseFrictionalForceMagnitude=off  SenseNormalForceMagnitude=off  SenseSeparationDistance=off  NormalTransitionRegionWidth=Trans  NormalTransitionRegionWidthUnits=m  FrictionType=SmoothStickSlip
  Spatial Contact Force5 : sm_lib/Forces and Torques/Spatial Contact Force  CoefficientOfDynamicFriction=DynamicF  CoefficientOfStaticFriction=StaticF  NormalDamping=Damp  NormalDampingUnits=N/(m/s)  NormalStiffness=Stiff  NormalStiffnessUnits=N/m  FrictionalCriticalVelocity=CriticalV  FrictionalCriticalVelocityUnits=m/s  ZeroCrossDetectContactStartAndEnd=off  SenseFrictionalForceMagnitude=off  SenseNormalForceMagnitude=off  SenseSeparationDistance=on  NormalTransitionRegionWidth=Trans  NormalTransitionRegionWidthUnits=m  FrictionType=SmoothStickSlip
  Simscape Bus1 : PMIOPort  Side=Left
  Spatial Contact Force1 : PMIOPort  Port=2  Side=Right
  LE_0.001 : Outport
  wires:
  PS-Simulink Converter1/1 -> Relational Operator/1
  Constant/1 -> Relational Operator/2
  Relational Operator/1 -> LE_0.001/1
  connections:
  Simscape Bus2/LConn3 -- Spatial Contact Force5/LConn1
  Spatial Contact Force3/LConn1 -- Simscape Bus2/LConn1
  Spatial Contact Force4/RConn1 -- Spatial Contact Force1/RConn1 -- Spatial Contact Force5/RConn1 -- Spatial Contact Force3/RConn1
  Simscape Bus2/RConn1 -- Simscape Bus1/RConn1
  Spatial Contact Force4/LConn1 -- Simscape Bus2/LConn2
  PS-Simulink Converter1/LConn1 -- Spatial Contact Force5/RConn2
